simulink model "seminar_simulink2"  (R2020b)
settings: Solver=VariableStepAuto  StartTime=0.0  StopTime=4  RelTol=1e-3
values from neighbouring files (symbols this model uses):
  b = 0.5    [seminar.m]
  c = 150    [seminar.m]
  J = 0.00156    [seminar.m]
  Km = 1    [seminar.m]
  Kv = 5.55e-7    (= 5.55e-07)    [seminar.m]
  omegav = 113    [seminar.m]
  qrm = 25.6e-6    (= 2.56e-05)    [seminar.m]
undefined symbols (not defined in the file or in its folder): Kr
settings Model: Creator=dominik  LastModifiedBy=dominik

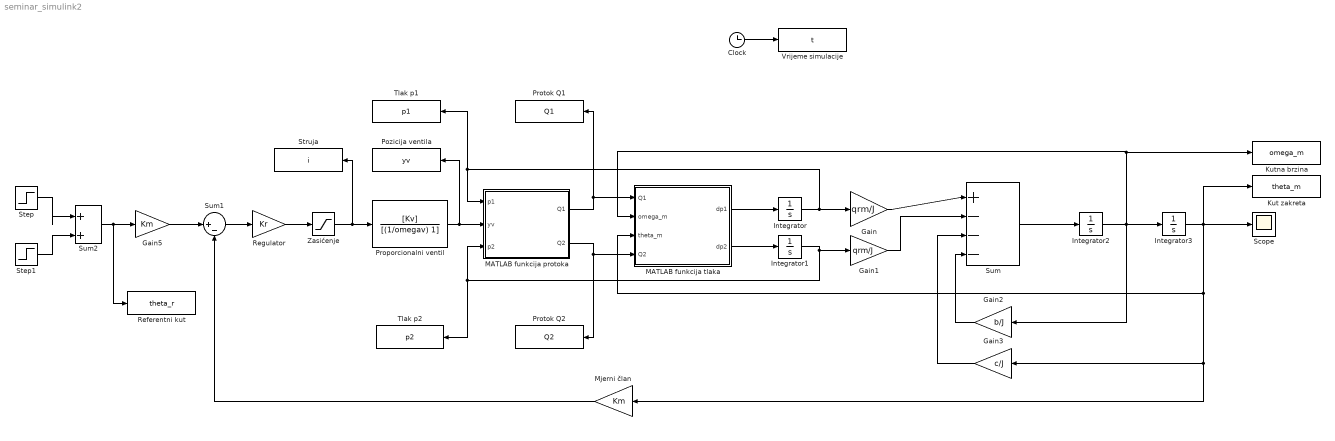
== system seminar_simulink2 ==
  Clock : Clock
  Gain : Gain  Gain=qrm/J
  Gain1 : Gain  Gain=qrm/J
  Gain2 : Gain  Gain=b/J
  Gain3 : Gain  Gain=c/J
  Gain5 : Gain  Gain=Km
  Integrator{,1..3} (4 alike) : Integrator
  Kut zakreta : ToWorkspace  VariableName=theta_m  SampleTime=-1
  Kutna brzina : ToWorkspace  VariableName=omega_m  SampleTime=-1
  MATLAB funkcija protoka : MATLAB Function  TreatAsAtomicUnit=on
  MATLAB funkcija tlaka : MATLAB Function  TreatAsAtomicUnit=on
  Mjerni član : Gain  Gain=Km
  Pozicija ventila : ToWorkspace  VariableName=yv  SampleTime=-1
  Proporcionalni ventil : TransferFcn  Numerator=[Kv]  Denominator=[(1/omegav) 1]
  Protok Q1 : ToWorkspace  VariableName=Q1  SampleTime=-1
  Protok Q2 : ToWorkspace  VariableName=Q2  SampleTime=-1
  Referentni kut : ToWorkspace  VariableName=theta_r  SampleTime=-1
  Regulator : Gain  Gain=Kr
  Scope : Scope
  Step : Step  Time=0  SampleTime=0
  Step1 : Step  Time=2  After=-2  SampleTime=0
  Struja : ToWorkspace  VariableName=i  SampleTime=-1
  Sum : Sum  Inputs=|+---
  Sum1 : Sum  Inputs=|+-
  Sum2 : Sum  Inputs=|++
  Tlak p1 : ToWorkspace  VariableName=p1  SampleTime=-1
  Tlak p2 : ToWorkspace  VariableName=p2  SampleTime=-1
  Vrijeme simulacije : ToWorkspace  VariableName=t  SampleTime=-1
  Zasićenje : Saturate  UpperLimit=10  LowerLimit=-10
  wires:
  MATLAB funkcija protoka/1(Q1) -> Protok Q1/1, MATLAB funkcija tlaka/1(Q1)
  MATLAB funkcija protoka/2(Q2) -> Protok Q2/1, MATLAB funkcija tlaka/4(Q2)
  Proporcionalni ventil/1 -> Pozicija ventila/1, MATLAB funkcija protoka/2(yv)
  MATLAB funkcija tlaka/1(dp1) -> Integrator/1
  MATLAB funkcija tlaka/2(dp2) -> Integrator1/1
  Integrator1/1 -> MATLAB funkcija protoka/3(p2), Tlak p2/1, Gain1/1
  Integrator/1 -> MATLAB funkcija protoka/1(p1), Tlak p1/1, Gain/1
  Gain/1 -> Sum/1
  Gain1/1 -> Sum/2
  Sum/1 -> Integrator2/1
  Integrator3/1 -> Kut zakreta/1, MATLAB funkcija tlaka/3(theta_m), Mjerni član/1, Gain3/1, Scope/1
  Gain2/1 -> Sum/4
  Gain3/1 -> Sum/3
  Integrator2/1 -> MATLAB funkcija tlaka/2(omega_m), Kutna brzina/1, Gain2/1, Integrator3/1
  Gain5/1 -> Sum1/1
  Mjerni član/1 -> Sum1/2
  Sum1/1 -> Regulator/1
  Step1/1 -> Sum2/2
  Step/1 -> Sum2/1
  Sum2/1 -> Referentni kut/1, Gain5/1
  Regulator/1 -> Zasićenje/1
  Zasićenje/1 -> Struja/1, Proporcionalni ventil/1
  Clock/1 -> Vrijeme simulacije/1

== matlab function seminar_simulink2/MATLAB funkcija protoka ==
  data: p1 input; Q1 output; yv input; p2 input; Q2 output
function [Q1, Q2] = protok(p1, yv, p2)

ps = 100e5;
pa = 1e5;

if yv >= 0
    Q1 = yv * sqrt(abs(ps - p1)) * sign(ps - p1);
    Q2 = -yv * sqrt(abs(p2 - pa)) * sign(p2 - pa);
else
    Q1 = yv * sqrt(abs(p1 - pa)) * sign(p1 - pa);
    Q2 = -yv * sqrt(abs(ps - p2)) * sign(ps - p2);
end

end

== matlab function seminar_simulink2/MATLAB funkcija tlaka ==
  data: Q1 input; dp1 output; omega_m input; theta_m input; Q2 input; dp2 output
function [dp1, dp2] = tlak(Q1, omega_m, theta_m, Q2)

qrm = 25.4e-6;
B = 1350e6;
V0 = 150e-6;

dp1 = (B/(V0 + qrm*theta_m) * (Q1 - qrm*omega_m));
dp2 = (B/(V0 - qrm*theta_m) * (Q2 + qrm*omega_m));

end
